simulink model "NDT_Localization"  (R2022a)
settings: Solver=FixedStepAuto  StartTime=0.0  StopTime=10.0  RelTol=1e-3
model workspace (MAT data in the model file):
  SL_ROS_VariableLengthArrays_MaxSizes : object (value not decoded)
undefined symbols (not defined in the file or in its folder): null
libraries: ros2lib x9, robotlib x8, simulink x1
(part 3 of 12)

== system NDT_Localization/observation_callback/check_localizer/If Action Subsystem/guess/extrapolate/lookupTransform/if_true/If Action Subsystem ==
  In1 : Inport
  Action Port : ActionPort  ActionPortLabel=else
  Out1 : Outport
  wires:
  In1/1 -> Out1/1

== system NDT_Localization/observation_callback/check_localizer/If Action Subsystem/guess/extrapolate/lookupTransform/if_true/If Action Subsystem1 ==
  cache : Inport
  Action Port : ActionPort  ActionPortLabel=if(u1 == u2)
  Constant : Constant  Commented=on  Value=null
  Constant1 : Constant  Value=true  OutDataTypeStr=boolean
  Constant2 : Constant  Value=false  OutDataTypeStr=boolean
  If : If  NumInputs=2  IfExpression=u1 ~= u2
  If Action Subsystem : Subsystem  TreatAsAtomicUnit=on
  If Action Subsystem1 : Subsystem  TreatAsAtomicUnit=on
  Merge : Merge
  out1 : Outport
  wires:
  Constant/1 -> If/2
  If/1 -> If Action Subsystem/Action
  If/2 -> If Action Subsystem1/Action
  Constant1/1 -> If Action Subsystem/1(In1)
  Constant2/1 -> If Action Subsystem1/1(In1)
  If Action Subsystem/1(Out1) -> Merge/1
  If Action Subsystem1/1(Out1) -> Merge/2
  Merge/1 -> out1/1
  cache/1 -> If/1

== system NDT_Localization/observation_callback/check_localizer/If Action Subsystem/guess/extrapolate/lookupTransform/if_true/getFrame ==
  target_id : Inport
  cache : Outport
  wires:
  target_id/1 -> cache/1

== system NDT_Localization/observation_callback/check_localizer/If Action Subsystem/guess/extrapolate/lookupTransform/if_true/getLatestTimestamp ==
  cache : Inport
  LatestTimestamp : Outport
  wires:
  cache/1 -> LatestTimestamp/1

== system NDT_Localization/observation_callback/check_localizer/If Action Subsystem/guess/extrapolate/lookupTransform/if_true/lookupFrameNumber ==
  target_frame : Inport
  Cast : DataTypeConversion  OutDataTypeStr=uint32  SaturateOnIntegerOverflow=off  RndMeth=Floor
  target_id : Outport
  wires:
  target_frame/1 -> Cast/1
  Cast/1 -> target_id/1

== system NDT_Localization/observation_callback/check_localizer/If Action Subsystem/guess/lookupTransform/if_true/If Action Subsystem1/If Action Subsystem ==
  In1 : Inport
  Action Port : ActionPort  ActionPortLabel=if(u1 ~= u2)
  Out1 : Outport
  wires:
  In1/1 -> Out1/1

== system NDT_Localization/observation_callback/check_localizer/If Action Subsystem/guess/lookupTransform/if_true/If Action Subsystem1/If Action Subsystem1 ==
  In1 : Inport
  Action Port : ActionPort  ActionPortLabel=else
  Out1 : Outport
  wires:
  In1/1 -> Out1/1

== system NDT_Localization/observation_callback/check_localizer/If Action Subsystem/register_measurement_impl/If Action Subsystem/If Action Subsystem/insert/If Action Subsystem ==
  ob_msg_data : Inport
  In2 : Inport  Port=2
  Action Port : ActionPort  ActionPortLabel=if(u1 <= u2)
  If : If  NumInputs=2  IfExpression=u1 ~= u2
  If Action Subsystem : Subsystem  TreatAsAtomicUnit=on
  If Action Subsystem1 : Subsystem  TreatAsAtomicUnit=on
  MATLAB Function : MATLAB Function  TreatAsAtomicUnit=on
  Merge : Merge
  Width : Width
  points : Outport
  Out2 : Outport  Port=2
  wires:
  ob_msg_data/1 -> MATLAB Function/1(msg)
  Merge/1 -> Out2/1
  If Action Subsystem/1(Out1) -> Merge/1
  If/1 -> If Action Subsystem/Action
  If/2 -> If Action Subsystem1/Action
  If Action Subsystem1/1(Out1) -> Merge/2
  In2/1 -> If/2
  Width/1 -> If/1
  MATLAB Function/1(points) -> Width/1, points/1

== system NDT_Localization/observation_callback/check_localizer/If Action Subsystem/register_measurement_impl/If Action Subsystem/If Action Subsystem/insert/If Action Subsystem1 ==
  Action Port : ActionPort  ActionPortLabel=else
  Constant : Constant  Value=0
  Out1 : Outport
  wires:
  Constant/1 -> Out1/1

== system NDT_Localization/observation_callback/check_localizer/If Action Subsystem/register_measurement_impl/If Action Subsystem/If Action Subsystem/solve/For Iterator Subsystem ==
  data : Inport
  myu : Inport  Port=2
  sigma : Inport  Port=3
  outlier_ratio : Inport  Port=4
  voxel_size_x : Inport  Port=5
  voxel_size_y : Inport  Port=6
  voxel_size_z : Inport  Port=7
  set_jacobian : Inport  Port=8
  set_gradient : Inport  Port=9
  set_hessian : Inport  Port=10
  point_hessian : Inport  Port=11
  Affine : MATLAB Function  TreatAsAtomicUnit=on
  Delay : Delay  DelayLength=1
  For Iterator : ForIterator  IterationSource=external
  For Iterator Subsystem : Subsystem  TreatAsAtomicUnit=on
  MATLAB Function : MATLAB Function  TreatAsAtomicUnit=on
  Width : Width
  gradient_jaco : Subsystem
  make_c_param : Subsystem
  make_d_param : Subsystem
  score : Subsystem
  score_out : Outport
  jacobian_out : Outport  Port=2
  hessian_out : Outport  Port=3
  wires:
  make_c_param/1(c1) -> make_d_param/1(c1)
  voxel_size_z/1 -> make_c_param/4(voxel_size_z)
  outlier_ratio/1 -> make_c_param/1(outlier_ratio)
  make_d_param/2(d2) -> For Iterator Subsystem/9(d2), gradient_jaco/9(d2), score/6(d2)
  voxel_size_y/1 -> make_c_param/3(voxel_size_y)
  make_c_param/2(c2) -> make_d_param/2(c2)
  voxel_size_x/1 -> make_c_param/2(voxel_size_x)
  make_d_param/1(d1) -> For Iterator Subsystem/8(d1), score/5(d1), gradient_jaco/8(d1)
  Width/1 -> For Iterator/1
  For Iterator/1 -> For Iterator Subsystem/3(i), gradient_jaco/3(index), MATLAB Function/2(index)
  MATLAB Function/1(pt) -> Affine/1(u)
  Affine/1(out) -> score/4(x), For Iterator Subsystem/4(data), gradient_jaco/4(data)
  sigma/1 -> For Iterator Subsystem/5(sigma), score/2(sigma), gradient_jaco/5(sigma)
  myu/1 -> gradient_jaco/6(myu), For Iterator Subsystem/6(myu), score/3(myu)
  score/1(p) -> score_out/1, Delay/1
  Delay/1 -> score/1(score)
  set_jacobian/1 -> gradient_jaco/1(set_jacobian)
  gradient_jaco/1(Out1) -> jacobian_out/1
  set_gradient/1 -> For Iterator Subsystem/2(set_gradient), gradient_jaco/2(set_gradient)
  set_hessian/1 -> For Iterator Subsystem/1(set_hessian)
  data/1 -> For Iterator Subsystem/7(x), gradient_jaco/7(x), MATLAB Function/1(data), Width/1
  point_hessian/1 -> For Iterator Subsystem/10(point_hessian)
  For Iterator Subsystem/1(Out1) -> hessian_out/1

== system NDT_Localization/observation_callback/check_localizer/If Action Subsystem/register_measurement_impl/If Action Subsystem/If Action Subsystem/solve/If Action Subsystem ==
  jacobian : Inport
  Action Port : ActionPort  ActionPortLabel=if(u1 <= u2)
  Bus Creator : BusCreator  Inputs=3
  iteration : Constant  Value=0  OutDataTypeStr=uint64
  termination_type.CONVERGENCE : Constant  Value=0  OutDataTypeStr=uint32
  Out1 : Outport
  wires:
  jacobian/1 -> Bus Creator/1  "dist"
  iteration/1 -> Bus Creator/3  "iter"
  termination_type.CONVERGENCE/1 -> Bus Creator/2  "termination_type"
  Bus Creator/1 -> Out1/1  "OptimizationSummary"

== system NDT_Localization/observation_callback/check_localizer/If Action Subsystem/register_measurement_impl/If Action Subsystem/If Action Subsystem/solve/If Action Subsystem1 ==
  problem : Inport
  jacobian : Inport  Port=2
  hessian : Inport  Port=3
  Max_iter : Inport  Port=4
  eig_pose : Inport  Port=5
  outlier_ratio : Inport  Port=6
  voxel_size_x : Inport  Port=7
  voxel_size_y : Inport  Port=8
  voxel_size_z : Inport  Port=9
  localizer_ptr : Inport  Port=10
  Action Port : ActionPort  ActionPortLabel=else
  Add : Sum
  Constant : Constant
  For Iterator Subsystem : Subsystem  TreatAsAtomicUnit=on
  summary : Outport
  eig_pose_result : Outport  Port=2
  wires:
  Max_iter/1 -> Add/1, For Iterator Subsystem/1(Max_iter)
  For Iterator Subsystem/1(summary) -> summary/1
  jacobian/1 -> For Iterator Subsystem/3(jacobian)
  hessian/1 -> For Iterator Subsystem/4(hessian)
  Add/1 -> For Iterator Subsystem/2(break_iter)
  Constant/1 -> Add/2
  problem/1 -> For Iterator Subsystem/5(problem)
  eig_pose/1 -> For Iterator Subsystem/6(eig_pose)
  outlier_ratio/1 -> For Iterator Subsystem/7(outlier_ratio)
  voxel_size_x/1 -> For Iterator Subsystem/8(voxel_size_x)
  voxel_size_y/1 -> For Iterator Subsystem/9(voxel_size_y)
  voxel_size_z/1 -> For Iterator Subsystem/10(voxel_size_z)
  For Iterator Subsystem/2(eig_pose_result) -> eig_pose_result/1
  localizer_ptr/1 -> For Iterator Subsystem/11(localizer_ptr)

== system NDT_Localization/observation_callback/check_localizer/If Action Subsystem/register_measurement_impl/If Action Subsystem/If Action Subsystem/solve/angle_params ==
  pose : Inport
  Bus Creator : BusCreator  Inputs=6
  If : If  NumInputs=2  IfExpression=u1 > u2
  If Action Subsystem : Subsystem  TreatAsAtomicUnit=on
  If Action Subsystem1 : Subsystem  TreatAsAtomicUnit=on
  If Action Subsystem2 : Subsystem  TreatAsAtomicUnit=on
  If Action Subsystem3 : Subsystem  TreatAsAtomicUnit=on
  If Action Subsystem4 : Subsystem  TreatAsAtomicUnit=on
  If Action Subsystem5 : Subsystem  TreatAsAtomicUnit=on
  If1 : If  NumInputs=2  IfExpression=u1 > u2
  If2 : If  NumInputs=2  IfExpression=u1 > u2
  MATLAB Function : MATLAB Function  TreatAsAtomicUnit=on
  Merge{,1..5} (6 alike) : Merge
  approx_thresh : Constant  Value=0.00010
  params : Outport
  wires:
  pose/1 -> MATLAB Function/1(u)
  MATLAB Function/1(x) -> If/2, If Action Subsystem1/1(x)
  MATLAB Function/3(z) -> If2/2, If Action Subsystem5/1(z)
  MATLAB Function/2(y) -> If Action Subsystem3/1(y), If1/2
  If Action Subsystem1/1(Out1) -> Merge/2
  If Action Subsystem1/2(Out2) -> Merge1/2
  If Action Subsystem3/1(Out1) -> Merge2/2
  If Action Subsystem3/2(Out2) -> Merge3/2
  If Action Subsystem5/1(Out1) -> Merge4/2
  If Action Subsystem5/2(Out2) -> Merge5/2
  approx_thresh/1 -> If2/1, If1/1, If/1
  If/1 -> If Action Subsystem/Action
  If/2 -> If Action Subsystem1/Action
  If1/1 -> If Action Subsystem2/Action
  If1/2 -> If Action Subsystem3/Action
  If2/2 -> If Action Subsystem5/Action
  If2/1 -> If Action Subsystem4/Action
  If Action Subsystem/1(Out1) -> Merge/1
  If Action Subsystem/2(Out2) -> Merge1/1
  If Action Subsystem2/1(Out1) -> Merge2/1
  If Action Subsystem2/2(Out2) -> Merge3/1
  If Action Subsystem4/1(Out1) -> Merge4/1
  If Action Subsystem4/2(Out2) -> Merge5/1
  Bus Creator/1 -> params/1
  Merge/1 -> Bus Creator/1  "cx"
  Merge1/1 -> Bus Creator/2  "sx"
  Merge2/1 -> Bus Creator/3  "cy"
  Merge3/1 -> Bus Creator/4  "sy"
  Merge4/1 -> Bus Creator/5  "cz"
  Merge5/1 -> Bus Creator/6  "sz"

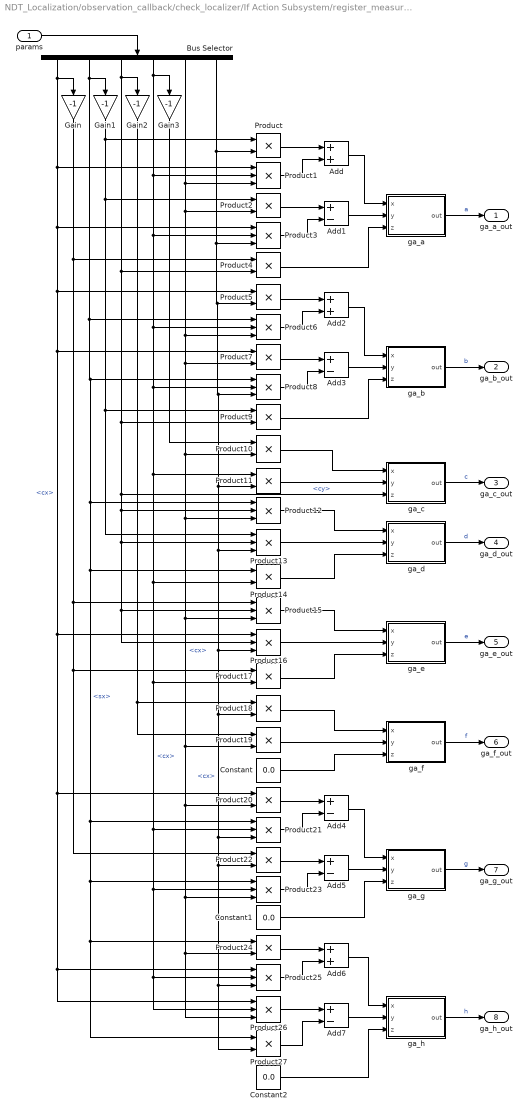
== system NDT_Localization/observation_callback/check_localizer/If Action Subsystem/register_measurement_impl/If Action Subsystem/If Action Subsystem/solve/gradient_angle ==
  params : Inport
  Add : Sum
  Add{1,3..5,7} (5 alike) : Sum  Inputs=+-
  Add2 : Sum
  Add6 : Sum
  Bus Selector : BusSelector  OutputSignals=cx,sx,cy,sy,cz,sz
  Constant : Constant  Value=0.0
  Constant1 : Constant  Value=0.0
  Constant2 : Constant  Value=0.0
  Gain{,1..3} (4 alike) : Gain  Gain=-1
  Product{,2,4..5,7,9..11,14,17..20,22,24,27} (16 alike) : Product
  Product{1,3,6,8,12..13,15..16,21,23,25..26} (12 alike) : Product  Inputs=3
  ga_a : MATLAB Function  TreatAsAtomicUnit=on
  ga_b : MATLAB Function  TreatAsAtomicUnit=on
  ga_c : MATLAB Function  TreatAsAtomicUnit=on
  ga_d : MATLAB Function  TreatAsAtomicUnit=on
  ga_e : MATLAB Function  TreatAsAtomicUnit=on
  ga_f : MATLAB Function  TreatAsAtomicUnit=on
  ga_g : MATLAB Function  TreatAsAtomicUnit=on
  ga_h : MATLAB Function  TreatAsAtomicUnit=on
  ga_a_out : Outport
  ga_b_out : Outport  Port=2
  ga_c_out : Outport  Port=3
  ga_d_out : Outport  Port=4
  ga_e_out : Outport  Port=5
  ga_f_out : Outport  Port=6
  ga_g_out : Outport  Port=7
  ga_h_out : Outport  Port=8
  wires:
  params/1 -> Bus Selector/1
  Bus Selector/1 -> Product1/1, Product16/1, Product25/1, Product26/1, Product20/1, Product7/1, Product5/1, Product3/1, Gain/1  "<cx>"
  Bus Selector/2 -> Product6/1, Product12/1, Product14/1, Product21/1, Product23/1, Product27/1, Product24/1, Product8/1, Gain1/1  "<sx>"
  Bus Selector/3 -> Product12/2, Product13/2, Product15/2, Product16/2, ga_c/3(z), Product9/2, Product4/2, Gain2/1  "<cy>"
  Bus Selector/4 -> Product11/1, Product14/2, Product17/2, Product21/2, Product25/2, Product26/2, Product23/2, Product8/2, Product6/2, Product3/2, Product1/2, Gain3/1  "<cx>"
  Bus Selector/5 -> Product6/3, Product10/2, Product12/3, Product15/3, Product19/2, Product20/2, Product23/3, Product26/3, Product24/2, Product7/2, Product2/2, Product1/3  "<cx>"
  Bus Selector/6 -> Product11/2, Product13/3, Product16/3, Product18/2, Product21/3, Product22/2, Product25/3, Product27/2, Product8/3, Product5/2, Product3/3, Product/2  "<cx>"
  Gain1/1 -> Product13/1, Product9/1, Product2/1, Product/1
  Product/1 -> Add/1
  Product1/1 -> Add/2
  Product2/1 -> Add1/1
  Add/1 -> ga_a/1(x)
  Add1/1 -> ga_a/2(y)
  Gain/1 -> Product15/1, Product17/1, Product22/1, Product4/1
  Product4/1 -> ga_a/3(z)
  Product3/1 -> Add1/2
  Product6/1 -> Add2/2
  Product7/1 -> Add3/1
  Product8/1 -> Add3/2
  Product5/1 -> Add2/1
  Add2/1 -> ga_b/1(x)
  Product9/1 -> ga_b/3(z)
  Add3/1 -> ga_b/2(y)
  Product11/1 -> ga_c/2(y)
  Product10/1 -> ga_c/1(x)
  Gain2/1 -> Product18/1, Product19/1
  Gain3/1 -> Product10/1
  Product13/1 -> ga_d/2(y)
  Product12/1 -> ga_d/1(x)
  Product14/1 -> ga_d/3(z)
  Product19/1 -> ga_f/2(y)
  Constant/1 -> ga_f/3(z)
  Product18/1 -> ga_f/1(x)
  Product16/1 -> ga_e/2(y)
  Product17/1 -> ga_e/3(z)
  Product15/1 -> ga_e/1(x)
  Product21/1 -> Add4/2
  Product22/1 -> Add5/1
  Product23/1 -> Add5/2
  Product20/1 -> Add4/1
  Add5/1 -> ga_g/2(y)
  Product25/1 -> Add6/2
  Product26/1 -> Add7/1
  Product27/1 -> Add7/2
  Product24/1 -> Add6/1
  Constant1/1 -> ga_g/3(z)
  Add4/1 -> ga_g/1(x)
  Add7/1 -> ga_h/2(y)
  Add6/1 -> ga_h/1(x)
  Constant2/1 -> ga_h/3(z)
  ga_a/1(out) -> ga_a_out/1  "a"
  ga_b/1(out) -> ga_b_out/1  "b"
  ga_c/1(out) -> ga_c_out/1  "c"
  ga_d/1(out) -> ga_d_out/1  "d"
  ga_e/1(out) -> ga_e_out/1  "e"
  ga_f/1(out) -> ga_f_out/1  "f"
  ga_g/1(out) -> ga_g_out/1  "g"
  ga_h/1(out) -> ga_h_out/1  "h"

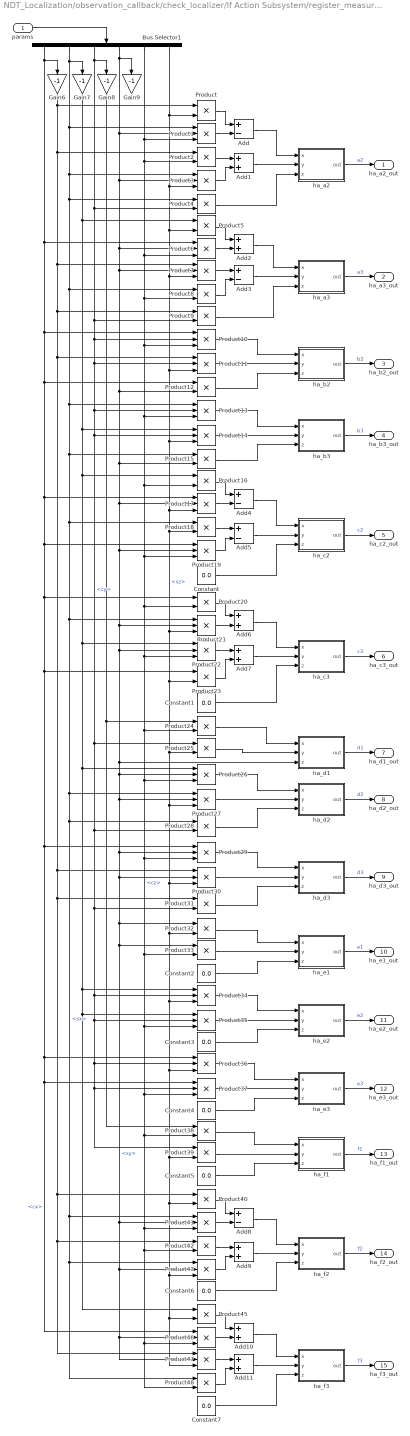
== system NDT_Localization/observation_callback/check_localizer/If Action Subsystem/register_measurement_impl/If Action Subsystem/If Action Subsystem/solve/hessian_angle ==
  params : Inport
  Add{,3..5,8} (5 alike) : Sum  Inputs=+-
  Add{1..2,6..7,9..11} (7 alike) : Sum
  Bus Selector1 : BusSelector  OutputSignals=cx,sx,cy,sy,cz,sz
  Constant{,1..7} (8 alike) : Constant  Value=0.0
  Gain{6..9} (4 alike) : Gain  Gain=-1
  Product{,2,4..5,8..9,12,15..16,18,20,23..25,28,31..33,38..40,42,45,48} (24 alike) : Product
  Product{1,3,6..7,10..11,13..14,17,19,21..22,26..27,29..30,34..37,41,43,46..47} (24 alike) : Product  Inputs=3
  ha_a2 : MATLAB Function  TreatAsAtomicUnit=on
  ha_a3 : MATLAB Function  TreatAsAtomicUnit=on
  ha_b2 : MATLAB Function  TreatAsAtomicUnit=on
  ha_b3 : MATLAB Function  TreatAsAtomicUnit=on
  ha_c2 : MATLAB Function  TreatAsAtomicUnit=on
  ha_c3 : MATLAB Function  TreatAsAtomicUnit=on
  ha_d1 : MATLAB Function  TreatAsAtomicUnit=on
  ha_d2 : MATLAB Function  TreatAsAtomicUnit=on
  ha_d3 : MATLAB Function  TreatAsAtomicUnit=on
  ha_e1 : MATLAB Function  TreatAsAtomicUnit=on
  ha_e2 : MATLAB Function  TreatAsAtomicUnit=on
  ha_e3 : MATLAB Function  TreatAsAtomicUnit=on
  ha_f1 : MATLAB Function  TreatAsAtomicUnit=on
  ha_f2 : MATLAB Function  TreatAsAtomicUnit=on
  ha_f3 : MATLAB Function  TreatAsAtomicUnit=on
  ha_a2_out : Outport
  ha_a3_out : Outport  Port=2
  ha_b2_out : Outport  Port=3
  ha_b3_out : Outport  Port=4
  ha_c2_out : Outport  Port=5
  ha_c3_out : Outport  Port=6
  ha_d1_out : Outport  Port=7
  ha_d2_out : Outport  Port=8
  ha_d3_out : Outport  Port=9
  ha_e1_out : Outport  Port=10
  ha_e2_out : Outport  Port=11
  ha_e3_out : Outport  Port=12
  ha_f1_out : Outport  Port=13
  ha_f2_out : Outport  Port=14
  ha_f3_out : Outport  Port=15
  wires:
  Bus Selector1/1 -> Product6/1, Product10/1, Product12/1, Product17/1, Product19/1, Product20/1, Product23/1, Product29/1, Product36/1, Product37/1, Product46/1, Gain6/1  "<cx>"
  Bus Selector1/3 -> Product4/2, Product9/2, Product10/2, Product11/2, Product13/2, Product14/2, Product25/1, Product28/2, Product31/2, Product34/2, Product35/2, Product36/2, Product37/2, Product39/1, Gain8/1  "<cy>"
  Bus Selector1/4 -> Product1/2, Product3/2, Product6/2, Product7/2, Product15/2, Product17/2, Product19/2, ha_d1/3(z), Product27/2, Product29/2, Product30/2, Product32/1, Product33/1, Product41/2, Product43/2, Product47/2, Product46/2, Product26/2, Product22/2, Product21/2, Product12/2, Gain9/1  "<sy>"
  params/1 -> Bus Selector1/1
  Bus Selector1/2 -> Product1/1, Product3/1, Product4/1, Product8/1, Product13/1, Product15/1, Product18/1, Product21/1, Product27/1, Product28/1, Product41/1, Product43/1, Product48/1, Gain7/1  "<sx>"
  Bus Selector1/5 -> Product1/3, Product2/2, Product6/3, Product8/2, Product10/3, Product13/3, Product16/2, Product19/3, Product20/2, Product22/3, Product24/2, Product26/3, Product29/3, Product33/2, Product35/3, Product37/3, Product38/2, Product41/3, Product42/2, Product46/3, Product48/2  "<cz>"
  Bus Selector1/6 -> Product/2, Product3/3, Product5/2, Product7/3, Product11/3, Product14/3, Product17/3, Product18/2, Product21/3, Product23/2, Product25/2, Product30/3, Product32/2, Product34/3, Product36/3, Product39/2, Product40/2, Product43/3, Product45/2, Product47/3, Product27/3  "<sz>"
  ha_a2/1(out) -> ha_a2_out/1  "a2"
  ha_a3/1(out) -> ha_a3_out/1  "a3"
  ha_b3/1(out) -> ha_b3_out/1  "b3"
  ha_b2/1(out) -> ha_b2_out/1  "b2"
  ha_c3/1(out) -> ha_c3_out/1  "c3"
  ha_c2/1(out) -> ha_c2_out/1  "c2"
  ha_d3/1(out) -> ha_d3_out/1  "d3"
  ha_d2/1(out) -> ha_d2_out/1  "d2"
  ha_d1/1(out) -> ha_d1_out/1  "d1"
  ha_e1/1(out) -> ha_e1_out/1  "e1"
  ha_e3/1(out) -> ha_e3_out/1  "e3"
  ha_e2/1(out) -> ha_e2_out/1  "e2"
  ha_f1/1(out) -> ha_f1_out/1  "f1"
  ha_f3/1(out) -> ha_f3_out/1  "f3"
  ha_f2/1(out) -> ha_f2_out/1  "f2"
  Product1/1 -> Add/2
  Product/1 -> Add/1
  Product2/1 -> Add1/1
  Product3/1 -> Add1/2
  Product4/1 -> ha_a2/3(z)
  Add1/1 -> ha_a2/2(y)
  Add/1 -> ha_a2/1(x)
  Product9/1 -> ha_a3/3(z)
  Add3/1 -> ha_a3/2(y)
  Product8/1 -> Add3/2
  Product7/1 -> Add3/1
  Product6/1 -> Add2/2
  Product5/1 -> Add2/1
  Add2/1 -> ha_a3/1(x)
  Product11/1 -> ha_b2/2(y)
  Product10/1 -> ha_b2/1(x)
  Product12/1 -> ha_b2/3(z)
  Product14/1 -> ha_b3/2(y)
  Product13/1 -> ha_b3/1(x)
  Product15/1 -> ha_b3/3(z)
  Product19/1 -> Add5/2
  Product18/1 -> Add5/1
  Product17/1 -> Add4/2
  Product16/1 -> Add4/1
  Product23/1 -> Add7/2
  Product22/1 -> Add7/1
  Product21/1 -> Add6/2
  Product20/1 -> Add6/1
  Add5/1 -> ha_c2/2(y)
  Constant/1 -> ha_c2/3(z)
  Add4/1 -> ha_c2/1(x)
  Add7/1 -> ha_c3/2(y)
  Constant1/1 -> ha_c3/3(z)
  Add6/1 -> ha_c3/1(x)
  Product25/1 -> ha_d1/2(y)
  Product24/1 -> ha_d1/1(x)
  Product27/1 -> ha_d2/2(y)
  Product28/1 -> ha_d2/3(z)
  Product26/1 -> ha_d2/1(x)
  Product30/1 -> ha_d3/2(y)
  Product29/1 -> ha_d3/1(x)
  Product31/1 -> ha_d3/3(z)
  Product33/1 -> ha_e1/2(y)
  Product32/1 -> ha_e1/1(x)
  Constant2/1 -> ha_e1/3(z)
  Product35/1 -> ha_e2/2(y)
  Product34/1 -> ha_e2/1(x)
  Constant3/1 -> ha_e2/3(z)
  Constant4/1 -> ha_e3/3(z)
  Product37/1 -> ha_e3/2(y)
  Product36/1 -> ha_e3/1(x)
  Constant5/1 -> ha_f1/3(z)
  Product38/1 -> ha_f1/1(x)
  Product39/1 -> ha_f1/2(y)
  Product42/1 -> Add9/1
  Product41/1 -> Add8/2
  Product46/1 -> Add10/2
  Product48/1 -> Add11/2
  Product43/1 -> Add9/2
  Product40/1 -> Add8/1
  Product47/1 -> Add11/1
  Product45/1 -> Add10/1
  Add9/1 -> ha_f2/2(y)
  Add11/1 -> ha_f3/2(y)
  Add10/1 -> ha_f3/1(x)
  Add8/1 -> ha_f2/1(x)
  Constant6/1 -> ha_f2/3(z)
  Constant7/1 -> ha_f3/3(z)
  Gain7/1 -> Product5/1, Product14/1, Product16/1, Product22/1, Product34/1, Product35/1, Product45/1, Product26/1
  Gain8/1 -> Product24/1, Product38/1
  Gain6/1 -> Product2/1, Product7/1, Product9/1, Product11/1, Product30/1, Product31/1, Product40/1, Product42/1, Product47/1, Product/1

== system NDT_Localization/observation_callback/check_localizer/If Action Subsystem/register_measurement_impl/If Action Subsystem/If Action Subsystem/solve/is_valid_probability ==
  u : Inport
  Constant : Constant  Value=0
  Constant1 : Constant
  Logical Operator : Logic  Operator=OR  Inputs=3  AllPortsSameDT=off  OutDataTypeStr=boolean
  MATLAB Function : MATLAB Function  TreatAsAtomicUnit=on
  Relational Operator : RelationalOperator  Operator=>  OutDataTypeStr=boolean  RndMeth=Simplest  InputSameDT=off
  Relational Operator1 : RelationalOperator  Operator=<  OutDataTypeStr=boolean  RndMeth=Simplest  InputSameDT=off
  Switch : Switch  Criteria=u2 > Threshold  SaturateOnIntegerOverflow=off  InputSameDT=off
  false : Constant  Value=0
  true : Constant
  Out1 : Outport
  wires:
  Switch/1 -> Out1/1
  false/1 -> Switch/1
  true/1 -> Switch/3
  u/1 -> MATLAB Function/1(u), Relational Operator1/1, Relational Operator/1
  Constant1/1 -> Relational Operator/2
  Constant/1 -> Relational Operator1/2
  Logical Operator/1 -> Switch/2
  Relational Operator/1 -> Logical Operator/2
  Relational Operator1/1 -> Logical Operator/3
  MATLAB Function/1(y) -> Logical Operator/1

== system NDT_Localization/map_callback/check_localizer/set_map/set_map_impl/insert/insert_/If Action Subsystem/While Iterator Subsystem/If Action Subsystem ==
  voxel_idx : Inport
  vx : Inport  Port=2
  <stamp> : Inport  Port=3
  Action Port : ActionPort  ActionPortLabel=if(u1 ~= 0)
  Bus Creator : BusCreator  Inputs=3
  Constant : Constant
  insert_res : Outport
  Out2 : Outport  Port=2
  wires:
  voxel_idx/1 -> Bus Creator/1
  vx/1 -> Bus Creator/2
  Bus Creator/1 -> insert_res/1  "insert_res"
  Constant/1 -> Out2/1
  <stamp>/1 -> Bus Creator/3

== system NDT_Localization/map_callback/check_localizer/set_map/set_map_impl/insert/insert_/If Action Subsystem/While Iterator Subsystem/If Action Subsystem1 ==
  Action Port : ActionPort  ActionPortLabel=else
  Constant : Constant  Value=0
  Out1 : Outport
  wires:
  Constant/1 -> Out1/1

== system NDT_Localization/map_callback/check_localizer/set_map/set_map_impl/insert/insert_/If Action Subsystem/While Iterator Subsystem/index ==
  pt : Inport
  Add{,1..8,10..14} (14 alike) : Sum  Inputs=+-
  Add9 : Sum  Inputs=3  OutDataTypeStr=uint32
  Divide3 : Product  Inputs=*/
  Divide4 : Product  Inputs=*/*
  FEPS : MATLAB Function  TreatAsAtomicUnit=on
  MATLAB Function : MATLAB Function  TreatAsAtomicUnit=on
  Math Function : Math  Operator=reciprocal
  Math Function1 : Math  Operator=reciprocal
  Math Function2 : Math  Operator=reciprocal
  Product{,1..4} (5 alike) : Product
  Rounding Function : Rounding
  Rounding Function1 : Rounding
  Rounding Function2 : Rounding
  Switch{,1..5} (6 alike) : Switch  Criteria=u2 > Threshold  SaturateOnIntegerOverflow=off  InputSameDT=off
  max_point.x : Constant  Value=130.0
  max_point.y : Constant  Value=130.0
  max_point.z : Constant  Value=3.0
  min_point.x : Constant  Value=-130.0
  min_point.y : Constant  Value=-130.0
  min_point.z : Constant  Value=-3.0
  voxel_size.x : Constant  Value=2.0
  voxel_size.y : Constant  Value=2.0
  voxel_size.z : Constant  Value=2.0
  idx : Outport
  wires:
  pt/1 -> MATLAB Function/1(u)
  Add13/1 -> Switch3/1, Add4/2, Add11/1
  Math Function/1 -> Product/2
  Switch1/1 -> Add2/1
  min_point.z/1 -> Add8/2, Switch4/3, Add6/2
  Product3/1 -> Add9/2
  min_point.y/1 -> Add5/2, Switch2/3, Add3/2, Add11/2
  voxel_size.z/1 -> Math Function2/1
  Add4/1 -> Switch3/2
  Divide4/1 -> Product4/2  "z_stride"
  voxel_size.y/1 -> Math Function1/1, Divide4/2
  FEPS/1(y) -> Add14/2, Add13/2, Add12/2
  voxel_size.x/1 -> Math Function/1, Divide3/2
  Add10/1 -> Divide3/1
  Add8/1 -> Product2/1
  Product2/1 -> Rounding Function2/1
  min_point.x/1 -> Add10/2, Add2/2, Switch/3, Add/2
  Add6/1 -> Switch4/2
  Add11/1 -> Divide4/1
  Add1/1 -> Switch1/2
  Product1/1 -> Rounding Function1/1
  Divide3/1 -> Divide4/3, Product3/2  "y_stride"
  Switch4/1 -> Switch5/3
  Switch3/1 -> Add5/1
  Product/1 -> Rounding Function/1
  Switch/1 -> Switch1/3
  Add/1 -> Switch/2
  Add14/1 -> Switch5/1, Add7/2
  Add5/1 -> Product1/1
  Add12/1 -> Add1/2, Add10/1, Switch1/1
  Switch2/1 -> Switch3/3
  Add3/1 -> Switch2/2
  Math Function1/1 -> Product1/2
  Add7/1 -> Switch5/2
  Product4/1 -> Add9/3
  Add2/1 -> Product/1
  Switch5/1 -> Add8/1
  max_point.x/1 -> Add12/1
  Math Function2/1 -> Product2/2
  max_point.y/1 -> Add13/1
  max_point.z/1 -> Add14/1
  Add9/1 -> idx/1
  MATLAB Function/2(y) -> Add3/1, Add4/1, Switch2/1
  MATLAB Function/1(x) -> Add/1, Add1/1, Switch/1
  MATLAB Function/3(z) -> Add6/1, Switch4/1, Add7/1
  Rounding Function/1 -> Add9/1  "idx"
  Rounding Function1/1 -> Product3/1  "jdx"
  Rounding Function2/1 -> Product4/1  "kdx"

== system NDT_Localization/map_callback/check_localizer/set_map/set_map_impl/insert/insert_/validate_pcl_map/check_fields/For Iterator Subsystem ==
  In1 : Inport
  <fields> : Inport  Port=2
  double_field_size : Inport  Port=3
  double_field_idx : Inport  Port=4
  Add : Sum  Inputs=+-
  Bus Selector : BusSelector  OutputSignals=datatype,offset,count
  Constant : Constant  Value=8  OutDataTypeStr=uint8
  Constant1 : Constant
  Delay : Delay  DelayLength=1
  For Iterator : ForIterator  IterationSource=external
  Logical Operator : Logic  Inputs=3  AllPortsSameDT=off  OutDataTypeStr=boolean
  Logical Operator1 : Logic  AllPortsSameDT=off  OutDataTypeStr=boolean
  Logical Operator2 : Logic  Operator=NOT  AllPortsSameDT=off  OutDataTypeStr=boolean
  Product : Product
  Relational Operator : RelationalOperator  Operator===  OutDataTypeStr=boolean  RndMeth=Simplest  InputSameDT=off
  Relational Operator1 : RelationalOperator  Operator===  OutDataTypeStr=boolean  RndMeth=Simplest  InputSameDT=off
  Relational Operator2 : RelationalOperator  Operator===  OutDataTypeStr=boolean  RndMeth=Simplest  InputSameDT=off
  Selector : Selector  InputPortWidth=16  IndexOptions=Starting index (port)  Indices=[1 3]  OutputSizes=1
  Out1 : Outport
  wires:
  In1/1 -> For Iterator/1
  For Iterator/1 -> Add/2, Selector/2  "index"
  <fields>/1 -> Selector/1
  Selector/1 -> Bus Selector/1  "field"
  Bus Selector/1 -> Relational Operator/1  "<datatype>"
  Bus Selector/2 -> Relational Operator1/1  "<offset>"
  Bus Selector/3 -> Relational Operator2/1  "<count>"
  Constant/1 -> Relational Operator/2
  Constant1/1 -> Relational Operator2/2
  Product/1 -> Relational Operator1/2
  Relational Operator/1 -> Logical Operator/1
  Relational Operator1/1 -> Logical Operator/2
  Relational Operator2/1 -> Logical Operator/3
  double_field_size/1 -> Product/2
  double_field_idx/1 -> Add/1
  Add/1 -> Product/1
  Logical Operator/1 -> Logical Operator1/2
  Delay/1 -> Logical Operator1/1
  Logical Operator1/1 -> Logical Operator2/1, Delay/1
  Logical Operator2/1 -> Out1/1

== system NDT_Localization/map_callback/check_localizer/set_map/set_map_impl/insert/insert_/validate_pcl_map/check_fields/If Action Subsystem ==
  Action Port : ActionPort  ActionPortLabel=if(u1 ~= 0)
  Constant : Constant  Value=0
  Out1 : Outport
  wires:
  Constant/1 -> Out1/1

== system NDT_Localization/map_callback/check_localizer/set_map/set_map_impl/insert/insert_/validate_pcl_map/check_fields/Subsystem ==
  <fields> : Inport
  double_field_size : Inport  Port=2
  Bus Selector : BusSelector  OutputSignals=datatype,offset,count
  Constant : Constant  Value=9
  Constant1 : Constant  Value=6  OutDataTypeStr=uint8
  Constant2 : Constant  Value=2  OutDataTypeStr=uint8
  Logical Operator : Logic  Operator=NAND  Inputs=3  AllPortsSameDT=off  OutDataTypeStr=boolean
  Product : Product
  Relational Operator : RelationalOperator  Operator===  OutDataTypeStr=boolean  RndMeth=Simplest  InputSameDT=off
  Relational Operator1 : RelationalOperator  Operator===  OutDataTypeStr=boolean  RndMeth=Simplest  InputSameDT=off
  Relational Operator2 : RelationalOperator  Operator===  OutDataTypeStr=boolean  RndMeth=Simplest  InputSameDT=off
  Selector : Selector  InputPortWidth=16  IndexOptions=Starting index (port)  Indices=[1 3]  OutputSizes=1
  Out1 : Outport
  wires:
  <fields>/1 -> Selector/1
  Constant/1 -> Product/1, Selector/2
  Selector/1 -> Bus Selector/1  "field"
  Bus Selector/1 -> Relational Operator/1  "<datatype>"
  Bus Selector/2 -> Relational Operator1/1  "<offset>"
  Bus Selector/3 -> Relational Operator2/1  "<count>"
  Constant1/1 -> Relational Operator/2
  Constant2/1 -> Relational Operator2/2
  Product/1 -> Relational Operator1/2
  double_field_size/1 -> Product/2
  Relational Operator/1 -> Logical Operator/1
  Relational Operator1/1 -> Logical Operator/2
  Relational Operator2/1 -> Logical Operator/3
  Logical Operator/1 -> Out1/1

== system NDT_Localization/map_callback/check_localizer/set_map/set_map_impl/insert/insert_/validate_pcl_map/check_fields/check_fields_name ==
  <fields> : Inport
  msg : Inport  Port=2
  Action Port : ActionPort  ActionPortLabel=else
  For Iterator Subsystem : Subsystem  TreatAsAtomicUnit=on
  For Iterator Subsystem1 : Subsystem  TreatAsAtomicUnit=on
  MATLAB Function : MATLAB Function  TreatAsAtomicUnit=on
  String Constant : StringConstant  String="\"x\""
  String Constant1 : StringConstant  String="\"y\""
  String Constant2 : StringConstant  String="\"z\""
  String Constant3 : StringConstant  String="\"icov_xx\""
  String Constant4 : StringConstant  String="\"icov_xy\""
  String Constant5 : StringConstant  String="\"icov_xz\""
  String Constant6 : StringConstant  String="\"icov_yy\""
  String Constant7 : StringConstant  String="\"icov_yz\""
  String Constant8 : StringConstant  String="\"icov_zz\""
  String Constant9 : StringConstant  String="\"cell_id\""
  Width : Width
  Out1 : Outport
  offset : Outport  Port=2
  ret : Outport  Port=3
  wires:
  Width/1 -> For Iterator Subsystem1/1(In2), For Iterator Subsystem/1(In1)
  <fields>/1 -> For Iterator Subsystem/2(fields), Width/1
  For Iterator Subsystem/1(name) -> For Iterator Subsystem1/2(name)
  String Constant/1 -> MATLAB Function/1(data)
  String Constant3/1 -> MATLAB Function/4(data3)
  String Constant6/1 -> MATLAB Function/7(data6)
  String Constant2/1 -> MATLAB Function/3(data2)
  String Constant4/1 -> MATLAB Function/5(data4)
  String Constant5/1 -> MATLAB Function/6(data5)
  String Constant7/1 -> MATLAB Function/8(data7)
  String Constant8/1 -> MATLAB Function/9(data8)
  String Constant1/1 -> MATLAB Function/2(data1)
  String Constant9/1 -> MATLAB Function/10(data9)
  MATLAB Function/1(names) -> For Iterator Subsystem1/3(names)
  For Iterator Subsystem1/1(Out1) -> Out1/1
  msg/1 -> For Iterator Subsystem1/4(msg)
  For Iterator Subsystem/2(offset) -> offset/1
  For Iterator Subsystem1/2(ret) -> ret/1

== system NDT_Localization/observation_callback/check_localizer/If Action Subsystem/guess/extrapolate/lookupTransform/if_true/If Action Subsystem1/If Action Subsystem ==
  In1 : Inport
  Action Port : ActionPort  ActionPortLabel=if(u1 ~= u2)
  Out1 : Outport
  wires:
  In1/1 -> Out1/1

== system NDT_Localization/observation_callback/check_localizer/If Action Subsystem/guess/extrapolate/lookupTransform/if_true/If Action Subsystem1/If Action Subsystem1 ==
  In1 : Inport
  Action Port : ActionPort  ActionPortLabel=else
  Out1 : Outport
  wires:
  In1/1 -> Out1/1

== system NDT_Localization/observation_callback/check_localizer/If Action Subsystem/register_measurement_impl/If Action Subsystem/If Action Subsystem/insert/If Action Subsystem/If Action Subsystem ==
  Action Port : ActionPort  ActionPortLabel=if(u1 ~= u2)
  Constant : Constant
  Out1 : Outport
  wires:
  Constant/1 -> Out1/1

== system NDT_Localization/observation_callback/check_localizer/If Action Subsystem/register_measurement_impl/If Action Subsystem/If Action Subsystem/insert/If Action Subsystem/If Action Subsystem1 ==
  Action Port : ActionPort  ActionPortLabel=else
  Constant : Constant  Value=0
  Out1 : Outport
  wires:
  Constant/1 -> Out1/1

== system NDT_Localization/observation_callback/check_localizer/If Action Subsystem/register_measurement_impl/If Action Subsystem/If Action Subsystem/solve/For Iterator Subsystem/For Iterator Subsystem ==
  set_hessian : Inport
  set_gradient : Inport  Port=2
  i : Inport  Port=3
  data : Inport  Port=4
  sigma : Inport  Port=5
  myu : Inport  Port=6
  x : Inport  Port=7
  d1 : Inport  Port=8
  d2 : Inport  Port=9
  point_hessian : Inport  Port=10
  Add : Sum  Inputs=+-
  Add1 : Sum  Inputs=+++
  Constant : Constant  Value=-2
  Divide1 : Product  Inputs=*/
  For Iterator : ForIterator  IterationSource=external
  MATLAB Function : MATLAB Function  TreatAsAtomicUnit=on
  MATLAB Function1 : MATLAB Function  TreatAsAtomicUnit=on
  Math Function : Math
  Math Function1 : Math  Operator=transpose
  Math Function2 : Math  Operator=reciprocal
  Product : Product  Inputs=4
  Product1 : Product  Inputs=3  Multiplication=Matrix(*)
  Product{4,6,8,10} (4 alike) : Product  Multiplication=Matrix(*)
  Product{2..3,5,7,9} (5 alike) : Product
  gradient_col_i : MATLAB Function  TreatAsAtomicUnit=on
  gradient_col_j : MATLAB Function  TreatAsAtomicUnit=on
  hessian_add : MATLAB Function  TreatAsAtomicUnit=on
  Out1 : Outport
  wires:
  Product3/1 -> Product8/2, Product4/2
  Product4/1 -> Product7/1
  Constant/1 -> Divide1/2
  set_gradient/1 -> gradient_col_j/2(gradient), gradient_col_i/2(gradient)
  hessian_add/1(hessian) -> Out1/1
  set_hessian/1 -> MATLAB Function/1(u), hessian_add/1("hessian ")
  i/1 -> hessian_add/2(index_i), gradient_col_i/1(index_i), MATLAB Function1/1(index_i)
  sigma/1 -> Math Function2/1
  Product/1 -> hessian_add/4(num)
  gradient_col_i/1(y) -> Product3/2
  data/1 -> Product10/1, Product6/1, Product4/1
  Add/1 -> Product1/3, Math Function1/1  "x-myu"
  d2/1 -> Divide1/1, Product/3  "d2"
  Product2/1 -> Math Function/1
  Divide1/1 -> Product2/1
  Math Function/1 -> Product/4
  Math Function1/1 -> Product1/1
  x/1 -> Add/1
  d1/1 -> Product/2  "d1"
  Product1/1 -> Product2/2
  myu/1 -> Add/2
  Math Function2/1 -> Product5/1, Product3/1, Product9/1, Product1/2  "inv_cov"
  MATLAB Function/1(y) -> For Iterator/1
  For Iterator/1 -> hessian_add/3(index_j), MATLAB Function1/2(index_j), gradient_col_j/1(index_j)
  Product5/1 -> Product6/2
  gradient_col_j/1(y) -> Product8/1, Product5/2
  Product6/1 -> Product7/2
  Product7/1 -> Add1/1
  Add1/1 -> Product/1
  Product8/1 -> Add1/3
  Product9/1 -> Product10/2
  Product10/1 -> Add1/2
  point_hessian/1 -> MATLAB Function1/3(point_hessian)
  MATLAB Function1/1(y) -> Product9/2

== system NDT_Localization/observation_callback/check_localizer/If Action Subsystem/register_measurement_impl/If Action Subsystem/If Action Subsystem/solve/For Iterator Subsystem/gradient_jaco ==
  set_jacobian : Inport
  set_gradient : Inport  Port=2
  index : Inport  Port=3
  data : Inport  Port=4
  sigma : Inport  Port=5
  myu : Inport  Port=6
  x : Inport  Port=7
  d1 : Inport  Port=8
  d2 : Inport  Port=9
  Add : Sum  Inputs=+-
  Constant : Constant  Value=-2
  Divide1 : Product  Inputs=*/
  Math Function : Math
  Math Function1 : Math  Operator=transpose
  Math Function2 : Math  Operator=reciprocal
  Product : Product  Inputs=4
  Product1 : Product  Inputs=3  Multiplication=Matrix(*)
  Product2 : Product
  Product3 : Product
  Product4 : Product  Multiplication=Matrix(*)
  gradient_col : MATLAB Function  TreatAsAtomicUnit=on
  jaco_add : MATLAB Function  TreatAsAtomicUnit=on
  Out1 : Outport
  wires:
  myu/1 -> Add/2
  Constant/1 -> Divide1/2
  Math Function1/1 -> Product1/1
  Divide1/1 -> Product2/1
  d2/1 -> Divide1/1, Product/3  "d2"
  Math Function2/1 -> Product3/2, Product1/2  "inv_cov"
  Product1/1 -> Product2/2
  d1/1 -> Product/2  "d1"
  x/1 -> Add/1
  Math Function/1 -> Product/4
  Product2/1 -> Math Function/1
  Add/1 -> Product1/3, Math Function1/1  "x-myu"
  sigma/1 -> Math Function2/1
  Product/1 -> jaco_add/3(num)
  index/1 -> jaco_add/2(index), gradient_col/1(index)
  jaco_add/1(jacobian) -> Out1/1
  set_jacobian/1 -> jaco_add/1("jacobian ")
  set_gradient/1 -> gradient_col/2(gradient)
  gradient_col/1(y) -> Product3/1
  data/1 -> Product4/1
  Product3/1 -> Product4/2
  Product4/1 -> Product/1

== system NDT_Localization/observation_callback/check_localizer/If Action Subsystem/register_measurement_impl/If Action Subsystem/If Action Subsystem/solve/For Iterator Subsystem/make_c_param ==
  outlier_ratio : Inport
  voxel_size_x : Inport  Port=2
  voxel_size_y : Inport  Port=3
  voxel_size_z : Inport  Port=4
  Constant : Constant
  Divide : Product  Inputs=*/
  Gain : Gain  Gain=10
  Product : Product  Inputs=3
  Subtract : Sum  Inputs=+-
  c1 : Outport
  c2 : Outport  Port=2
  wires:
  Constant/1 -> Subtract/1
  outlier_ratio/1 -> Divide/1, Subtract/2
  Subtract/1 -> Gain/1
  Gain/1 -> c1/1
  Product/1 -> Divide/2
  Divide/1 -> c2/1
  voxel_size_y/1 -> Product/2
  voxel_size_z/1 -> Product/3
  voxel_size_x/1 -> Product/1

== system NDT_Localization/observation_callback/check_localizer/If Action Subsystem/register_measurement_impl/If Action Subsystem/If Action Subsystem/solve/For Iterator Subsystem/make_d_param ==
  c1 : Inport
  c2 : Inport  Port=2
  Add1 : Sum
  Add2 : Sum  Inputs=-+
  Add3 : Sum
  Add4 : Sum  Inputs=+-
  Constant : Constant  Value=-2
  Constant1 : Constant  Value=-0.5
  Divide : Product  Inputs=*/
  Math Function{3..4,6..7} (4 alike) : Math  Operator=log
  Math Function5 : Math
  Product3 : Product
  Product4 : Product
  d1 : Outport
  d2 : Outport  Port=2
  wires:
  Add2/1 -> Divide/2, d1/1  "d1"
  Math Function4/1 -> Add4/1, Add2/2  "-d3"
  Product4/1 -> Add3/1
  Add3/1 -> Math Function6/1
  c1/1 -> Product4/1, Add1/1
  Constant/1 -> Product3/2
  Constant1/1 -> Math Function5/1
  Product3/1 -> d2/1  "d2"
  Math Function5/1 -> Product4/2
  Math Function7/1 -> Product3/1
  Divide/1 -> Math Function7/1
  Math Function6/1 -> Add4/2
  c2/1 -> Add3/2, Math Function4/1, Add1/2
  Add4/1 -> Divide/1
  Add1/1 -> Math Function3/1
  Math Function3/1 -> Add2/1

== system NDT_Localization/observation_callback/check_localizer/If Action Subsystem/register_measurement_impl/If Action Subsystem/If Action Subsystem/solve/For Iterator Subsystem/score ==
  score : Inport
  sigma : Inport  Port=2
  myu : Inport  Port=3
  x : Inport  Port=4
  d1 : Inport  Port=5
  d2 : Inport  Port=6
  Add : Sum  Inputs=+-
  Add1 : Sum
  Constant : Constant  Value=-2
  Divide1 : Product  Inputs=*/
  Gain : Gain  Gain=-1
  Math Function : Math
  Math Function1 : Math  Operator=transpose
  Math Function2 : Math  Operator=reciprocal
  Product : Product
  Product1 : Product  Inputs=3  Multiplication=Matrix(*)
  Product2 : Product
  p : Outport
  wires:
  sigma/1 -> Math Function2/1
  Math Function/1 -> Product/2
  Gain/1 -> Product/1  "-d1"
  myu/1 -> Add/2
  x/1 -> Add/1
  Product2/1 -> Math Function/1
  Add/1 -> Product1/3, Math Function1/1  "x-myu"
  Product/1 -> Add1/2
  Math Function1/1 -> Product1/1
  Product1/1 -> Product2/2
  Math Function2/1 -> Product1/2
  Constant/1 -> Divide1/2
  Divide1/1 -> Product2/1
  d2/1 -> Divide1/1  "d2"
  d1/1 -> Gain/1
  Add1/1 -> p/1
  score/1 -> Add1/1

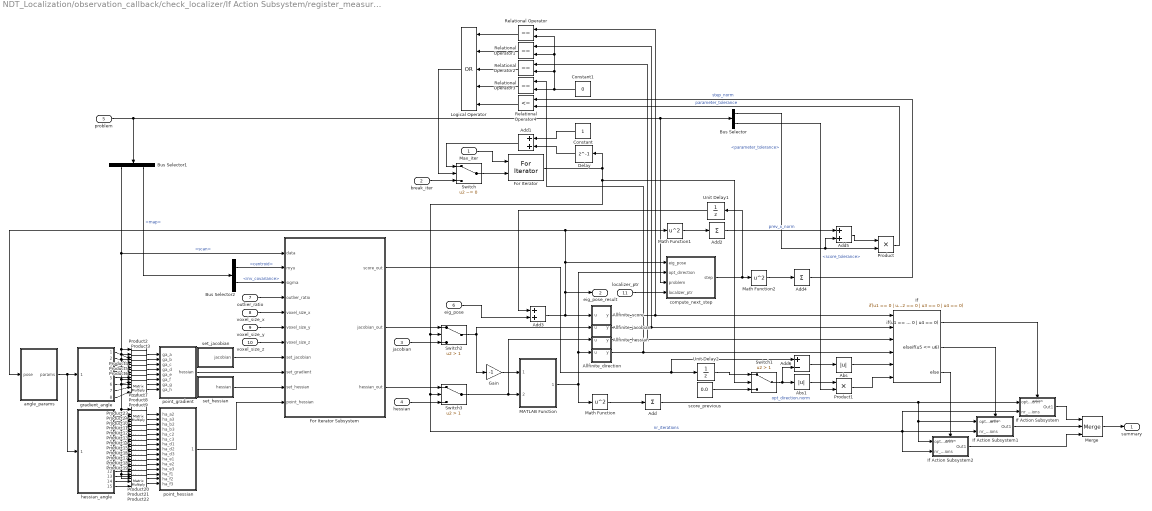
== system NDT_Localization/observation_callback/check_localizer/If Action Subsystem/register_measurement_impl/If Action Subsystem/If Action Subsystem/solve/If Action Subsystem1/For Iterator Subsystem ==
  Max_iter : Inport
  break_iter : Inport  Port=2
  jacobian : Inport  Port=3
  hessian : Inport  Port=4
  problem : Inport  Port=5
  eig_pose : Inport  Port=6
  outlier_ratio : Inport  Port=7
  voxel_size_x : Inport  Port=8
  voxel_size_y : Inport  Port=9
  voxel_size_z : Inport  Port=10
  localizer_ptr : Inport  Port=11
  Abs : Abs  SaturateOnIntegerOverflow=off
  Abs1 : Abs  SaturateOnIntegerOverflow=off
  Add : Sum  Inputs=+
  Add1 : Sum
  Add2 : Sum  Inputs=+
  Add3 : Sum
  Add4 : Sum  Inputs=+
  Add5 : Sum
  Add6 : Sum  Inputs=+-
  Allfinite_direction : MATLAB Function  TreatAsAtomicUnit=on
  Allfinite_hessian : MATLAB Function  TreatAsAtomicUnit=on
  Allfinite_jacobian : MATLAB Function  TreatAsAtomicUnit=on
  Allfinite_score : MATLAB Function  TreatAsAtomicUnit=on
  Bus Selector : BusSelector  OutputSignals=optimizer_options.parameter_tolerance,optimizer_options.score_tolerance
  Bus Selector1 : BusSelector  OutputSignals=scan,map
  Bus Selector2 : BusSelector  OutputSignals=vx.centroid,vx.inv_covariance
  Constant : Constant
  Constant1 : Constant  Value=0
  Delay : Delay  DelayLength=1
  For Iterator : ForIterator  IterationSource=external  ExternalIncrement=on
  For Iterator Subsystem : Subsystem  TreatAsAtomicUnit=on
  Gain : Gain  Gain=-1
  If : If  NumInputs=6  IfExpression=u1 == 0 | u2 == 0 | u3 == 0 | u4 == 0  ElseIfExpressions=u5 <= u6
  If Action Subsystem : Subsystem  TreatAsAtomicUnit=on
  If Action Subsystem1 : Subsystem  TreatAsAtomicUnit=on
  If Action Subsystem2 : Subsystem  TreatAsAtomicUnit=on
  Logical Operator : Logic  Operator=OR  Inputs=5  AllPortsSameDT=off  OutDataTypeStr=boolean
  MATLAB Function : MATLAB Function  TreatAsAtomicUnit=on
  Math Function : Math  Operator=square
  Math Function1 : Math  Operator=square
  Math Function2 : Math  Operator=square
  Merge : Merge  Inputs=3
  Product : Product
  Product1 : Product
  Product{2..24} (23 alike) : Product  Multiplication=Matrix(*)
  Relational Operator{,1..3} (4 alike) : RelationalOperator  Operator===  OutDataTypeStr=boolean  RndMeth=Simplest  InputSameDT=off
  Relational Operator4 : RelationalOperator  Operator=<=  OutDataTypeStr=boolean  RndMeth=Simplest  InputSameDT=off
  Switch : Switch  Criteria=u2 ~= 0  SaturateOnIntegerOverflow=off  InputSameDT=off
  Switch1 : Switch  Criteria=u2 > Threshold  Threshold=1  SaturateOnIntegerOverflow=off  InputSameDT=off
  Switch2 : Switch  Criteria=u2 > Threshold  Threshold=1  SaturateOnIntegerOverflow=off  InputSameDT=off
  Switch3 : Switch  Criteria=u2 > Threshold  Threshold=1  SaturateOnIntegerOverflow=off  InputSameDT=off
  Unit Delay1 : UnitDelay  SampleTime=-1  HasFrameUpgradeWarning=on
  Unit Delay2 : UnitDelay  SampleTime=-1  HasFrameUpgradeWarning=on
  angle_params : Subsystem
  compute_next_step : Subsystem
  gradient_angle : Subsystem
  hessian_angle : Subsystem
  point_gradient : MATLAB Function  TreatAsAtomicUnit=on
  point_hessian : MATLAB Function  TreatAsAtomicUnit=on
  score_previous : Constant  Value=0.0
  set_hessian : MATLAB Function  TreatAsAtomicUnit=on
  set_jacobian : MATLAB Function  TreatAsAtomicUnit=on
  summary : Outport
  eig_pose_result : Outport  Port=2
  wires:
  Max_iter/1 -> For Iterator/1
  Gain/1 -> MATLAB Function/1(jacobian)
  Switch3/1 -> MATLAB Function/2(hessian), Allfinite_hessian/1(u)
  MATLAB Function/1(opt_direction) -> Math Function/1, compute_next_step/2(opt_direction), Allfinite_direction/1(u)
  If/2 -> If Action Subsystem1/Action
  If/1 -> If Action Subsystem/Action
  If Action Subsystem/1(Out1) -> Merge/1
  Merge/1 -> summary/1
  If Action Subsystem1/1(Out1) -> Merge/2
  For Iterator/1 -> Delay/1, If Action Subsystem/2(nr_iterations), If Action Subsystem2/2(nr_iterations), If Action Subsystem1/2(nr_iterations), Switch3/2, Switch2/2, Switch1/2  "nr_iterations"
  Math Function/1 -> Add/1
  Add/1 -> If Action Subsystem2/1(opt_direction.norm), If Action Subsystem1/1(opt_direction.norm), If Action Subsystem/1(opt_direction.norm)  "opt_direction.norm"
  Allfinite_score/1(y) -> Relational Operator/1, If/1
  Allfinite_jacobian/1(y) -> Relational Operator1/1, If/2
  Allfinite_hessian/1(y) -> Relational Operator2/1, If/3
  Allfinite_direction/1(y) -> If/4, Relational Operator3/1
  Switch/1 -> For Iterator/2
  break_iter/1 -> Switch/3
  Add1/1 -> Switch/1
  Logical Operator/1 -> Switch/2
  Constant/1 -> Add1/1
  Delay/1 -> Add1/2
  Relational Operator/1 -> Logical Operator/1
  Relational Operator1/1 -> Logical Operator/2
  Relational Operator2/1 -> Logical Operator/3
  Relational Operator3/1 -> Logical Operator/4
  Constant1/1 -> Relational Operator2/2, Relational Operator1/2, Relational Operator/2, Relational Operator3/2
  Math Function1/1 -> Add2/1
  Add2/1 -> Add5/1  "prev_x_norm"
  compute_next_step/1(step) -> Unit Delay1/1, Math Function2/1
  Unit Delay1/1 -> Add3/1
  Bus Selector/1 -> Product/2, Add5/2  "<parameter_tolerance>"
  Add4/1 -> Relational Operator4/1  "step_norm"
  Math Function2/1 -> Add4/1
  Relational Operator4/1 -> Logical Operator/5
  Product/1 -> Relational Operator4/2  "parameter_tolerance"
  Add5/1 -> Product/1
  If Action Subsystem2/1(Out1) -> Merge/3
  If/3 -> If Action Subsystem2/Action
  Abs/1 -> If/5
  Product1/1 -> If/6
  Add6/1 -> Abs/1
  Abs1/1 -> Product1/1
  eig_pose/1 -> Add3/2
  Bus Selector/2 -> Product1/2  "<score_tolerance>"
  Switch1/1 -> Abs1/1, Add6/2
  Unit Delay2/1 -> Switch1/1
  score_previous/1 -> Switch1/3
  Add3/1 -> eig_pose_result/1, Math Function1/1, angle_params/1(pose), compute_next_step/1(eig_pose), Allfinite_score/1(u)
  Product10/1 -> point_hessian/3(ha_b2)
  gradient_angle/8(ga_h_out) -> Product9/2
  Product18/1 -> point_hessian/11(ha_e2)
  Product8/1 -> point_gradient/7(ga_g)
  Product22/1 -> point_hessian/15(ha_f3)
  point_gradient/1(hessian) -> For Iterator Subsystem/9(set_gradient)
  angle_params/1(params) -> hessian_angle/1(params), gradient_angle/1(params)
  hessian_angle/9(ha_d3_out) -> Product16/2
  Bus Selector2/2 -> For Iterator Subsystem/3(sigma)  "<inv_covariance>"
  hessian_angle/14(ha_f2_out) -> Product21/2
  Product17/1 -> point_hessian/10(ha_e1)
  Product3/1 -> point_gradient/2(ga_b)
  Product16/1 -> point_hessian/9(ha_d3)
  hessian_angle/15(ha_f3_out) -> Product22/2
  Product6/1 -> point_gradient/5(ga_e)
  Bus Selector1/2 -> Bus Selector2/1  "<map>"
  outlier_ratio/1 -> For Iterator Subsystem/4(outlier_ratio)
  gradient_angle/4(ga_d_out) -> Product5/2
  hessian_angle/11(ha_e2_out) -> Product18/2
  gradient_angle/2(ga_b_out) -> Product3/2
  Product14/1 -> point_hessian/7(ha_d1)
  Product15/1 -> point_hessian/8(ha_d2)
  hessian_angle/2(ha_a3_out) -> Product24/2
  hessian_angle/10(ha_e1_out) -> Product17/2
  hessian_angle/3(ha_b2_out) -> Product10/2
  point_hessian/1(hessian) -> For Iterator Subsystem/11(point_hessian)
  Product19/1 -> point_hessian/12(ha_e3)
  set_jacobian/1(jacobian) -> For Iterator Subsystem/8(set_jacobian)
  hessian_angle/8(ha_d2_out) -> Product15/2
  hessian_angle/6(ha_c3_out) -> Product13/2
  Product11/1 -> point_hessian/4(ha_b3)
  Product13/1 -> point_hessian/6(ha_c3)
  Product9/1 -> point_gradient/8(ga_h)
  hessian_angle/1(ha_a2_out) -> Product23/2
  Product24/1 -> point_hessian/2(ha_a3)
  hessian_angle/4(ha_b3_out) -> Product11/2
  Product5/1 -> point_gradient/4(ga_d)
  gradient_angle/7(ga_g_out) -> Product8/2
  Product2/1 -> point_gradient/1(ga_a)
  Product20/1 -> point_hessian/13(ha_f1)
  gradient_angle/6(ga_f_out) -> Product7/2
  set_hessian/1(hessian) -> For Iterator Subsystem/10(set_hessian)
  Product12/1 -> point_hessian/5(ha_c2)
  gradient_angle/1(ga_a_out) -> Product2/2
  Product7/1 -> point_gradient/6(ga_f)
  hessian_angle/7(ha_d1_out) -> Product14/2
  voxel_size_z/1 -> For Iterator Subsystem/7(voxel_size_z)
  Product21/1 -> point_hessian/14(ha_f2)
  hessian_angle/13(ha_f1_out) -> Product20/2
  voxel_size_y/1 -> For Iterator Subsystem/6(voxel_size_y)
  Bus Selector1/1 -> For Iterator Subsystem/1(data), Product2/1, Product3/1, Product4/1, Product5/1, Product6/1, Product7/1, Product8/1, Product9/1, Product23/1, Product24/1, Product10/1, Product11/1, Product12/1, Product13/1, Product14/1, Product15/1, Product16/1, Product17/1, Product18/1, Product19/1, Product20/1, Product21/1, Product22/1  "<scan>"
  hessian_angle/5(ha_c2_out) -> Product12/2
  hessian_angle/12(ha_e3_out) -> Product19/2
  voxel_size_x/1 -> For Iterator Subsystem/5(voxel_size_x)
  Product23/1 -> point_hessian/1(ha_a2)
  problem/1 -> compute_next_step/3(problem), Bus Selector/1, Bus Selector1/1
  Product4/1 -> point_gradient/3(ga_c)
  Bus Selector2/1 -> For Iterator Subsystem/2(myu)  "<centroid>"
  gradient_angle/3(ga_c_out) -> Product4/2
  gradient_angle/5(ga_e_out) -> Product6/2
  For Iterator Subsystem/1(score_out) -> Unit Delay2/1, Add6/1
  Switch2/1 -> Allfinite_jacobian/1(u), Gain/1
  jacobian/1 -> Switch2/3
  hessian/1 -> Switch3/3
  For Iterator Subsystem/2(jacobian_out) -> Switch2/1
  For Iterator Subsystem/3(hessian_out) -> Switch3/1
  localizer_ptr/1 -> compute_next_step/4(localizer_ptr)

== system NDT_Localization/observation_callback/check_localizer/If Action Subsystem/register_measurement_impl/If Action Subsystem/If Action Subsystem/solve/angle_params/If Action Subsystem ==
  Action Port : ActionPort  ActionPortLabel=if(u1 > u2)
  Constant : Constant
  Constant1 : Constant  Value=0
  Out1 : Outport
  Out2 : Outport  Port=2
  wires:
  Constant/1 -> Out1/1
  Constant1/1 -> Out2/1

== system NDT_Localization/observation_callback/check_localizer/If Action Subsystem/register_measurement_impl/If Action Subsystem/If Action Subsystem/solve/angle_params/If Action Subsystem1 ==
  x : Inport
  Action Port : ActionPort  ActionPortLabel=else
  Trigonometric Function : Trigonometry  Operator=cos
  Trigonometric Function1 : Trigonometry
  Out1 : Outport
  Out2 : Outport  Port=2
  wires:
  x/1 -> Trigonometric Function1/1, Trigonometric Function/1
  Trigonometric Function1/1 -> Out2/1
  Trigonometric Function/1 -> Out1/1

== system NDT_Localization/observation_callback/check_localizer/If Action Subsystem/register_measurement_impl/If Action Subsystem/If Action Subsystem/solve/angle_params/If Action Subsystem2 ==
  Action Port : ActionPort  ActionPortLabel=if(u1 > u2)
  Constant : Constant
  Constant1 : Constant  Value=0
  Out1 : Outport
  Out2 : Outport  Port=2
  wires:
  Constant/1 -> Out1/1
  Constant1/1 -> Out2/1
